simulink model "p1"  (R2017b)
settings: Solver=FixedStepAuto  StartTime=0.0  StopTime=10.0  FixedStep=0.01  RelTol=1e-3
undefined symbols (not defined in the file): a, b, c, K
settings Model: Creator=Soutrik  LastModifiedBy=Soutrik

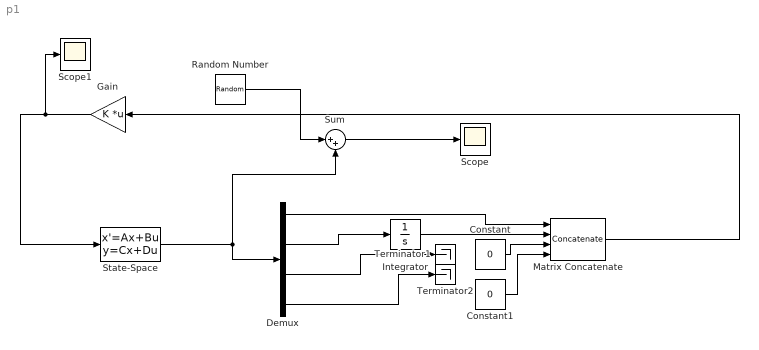
== system p1 ==
  Constant : Constant  Value=0
  Constant1 : Constant  Value=0
  Demux : Demux
  Gain : Gain  Gain=K  Multiplication=Matrix(K*u)
  Integrator : Integrator
  Matrix Concatenate : Concatenate  NumInputs=4  Mode=Multidimensional array  ConcatenateDimension=2
  Random Number : RandomNumber  Variance=[0.00001, 0.00001, 0.0001, 0.0001]  Seed=[1 2 3 4]  SampleTime=0.01
  Scope : Scope
  Scope1 : Scope
  State-Space : StateSpace  A=a  B=b  C=c  D=zeros(4,2)  InitialCondition=[0.05, 0, 0, 0]
  Sum : Sum  Inputs=|++
  Terminator1 : Terminator
  Terminator2 : Terminator
  wires:
  Random Number/1 -> Sum/1
  State-Space/1 -> Sum/2, Demux/1
  Sum/1 -> Scope/1
  Gain/1 -> Scope1/1, State-Space/1
  Demux/2 -> Integrator/1
  Demux/3 -> Terminator1/1
  Demux/4 -> Terminator2/1
  Demux/1 -> Matrix Concatenate/1
  Integrator/1 -> Matrix Concatenate/2
  Matrix Concatenate/1 -> Gain/1
  Constant/1 -> Matrix Concatenate/3
  Constant1/1 -> Matrix Concatenate/4
